simulink model "CarWashSimulinkSimulator"  (R2021b)
settings: Solver=FixedStepDiscrete  StartTime=0.0  StopTime=inf  RelTol=1e-3
model workspace (MAT data in the model file):
  SoapLevel = Simulink.Parameter
  SoapLevel.Value = 100
  SoapLevel.DataType = 'int8'
  SoapLevel.Min = 0
  SoapLevel.Max = 100
  SoapLevel.Complexity = 'real'
  SoapLevel.Dimensions = [1 1]
  UltraShineLevel = Simulink.Parameter
  UltraShineLevel.Value = 100
  UltraShineLevel.DataType = 'int8'
  UltraShineLevel.Min = 0
  UltraShineLevel.Max = 100
  UltraShineLevel.Complexity = 'real'
  UltraShineLevel.Dimensions = [1 1]
  WashType = 'standard'
  WaterPumpStatus = 1
  WaxLevel = Simulink.Parameter
  WaxLevel.Value = 1
  WaxLevel.DataType = 'double'
  WaxLevel.Min = 0
  WaxLevel.Max = 100
  WaxLevel.Complexity = 'real'
  WaxLevel.Dimensions = [1 1]
settings Model: Creator=Daniel Hernandez  LastModifiedBy=Daniel Hernandez

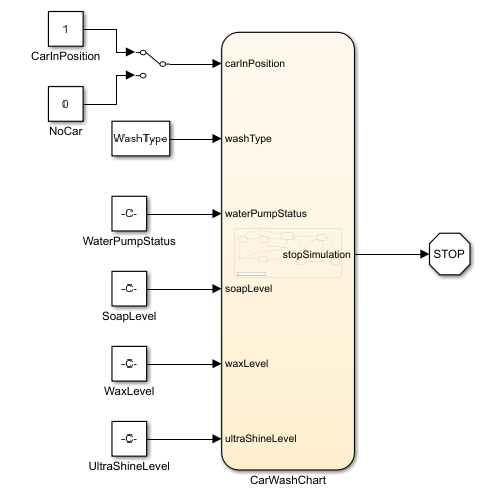
[thumbnail: Simulink's stored preview of the top-level diagram]
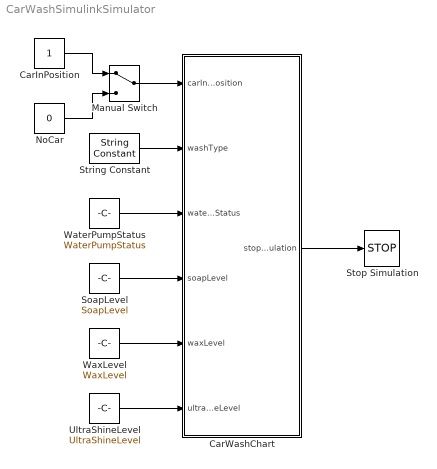
== system CarWashSimulinkSimulator ==
  CarInPosition : Constant
  CarWashChart : Stateflow chart  TreatAsAtomicUnit=on
  Manual Switch : ManualSwitch
  NoCar : Constant  Value=0
  SoapLevel : Constant  Value=SoapLevel
  Stop Simulation : Stop
  String Constant : StringConstant  String=WashType
  UltraShineLevel : Constant  Value=UltraShineLevel
  WaterPumpStatus : Constant  Value=WaterPumpStatus
  WaxLevel : Constant  Value=WaxLevel
  wires:
  CarInPosition/1 -> Manual Switch/1
  NoCar/1 -> Manual Switch/2
  Manual Switch/1 -> CarWashChart/1(carInPosition)
  CarWashChart/1(stopSimulation) -> Stop Simulation/1
  String Constant/1 -> CarWashChart/2(washType)
  WaterPumpStatus/1 -> CarWashChart/3(waterPumpStatus)
  SoapLevel/1 -> CarWashChart/4(soapLevel)
  WaxLevel/1 -> CarWashChart/5(waxLevel)
  UltraShineLevel/1 -> CarWashChart/6(ultraShineLevel)

== stateflow chart CarWashSimulinkSimulator/CarWashChart ==
  state AppInterface
    state Idle
    state Exiting
      ex:
      stopSimulation = 1
    state Ready
    state SprayingWater
    state Drying
    state Foaming
    state Waxing
    state Polishing
    state ValidationFailed
    (default) -> Idle
    Ready -> Exiting [order 2] : after(10,sec)
    Exiting -> Idle
    ValidationFailed -> Exiting
    (junction 26) -> Exiting [order 1] : [washType=='quick']
    (junction 30) -> Exiting [order 4]
    Drying -> Exiting : after(5,sec)
    Idle -> Ready [order 1] : after(1,sec)
    Ready -> (junction 25) [order 1] : [carInPosition == true]
    (junction 25) -> SprayingWater [order 1] : [washType=='quick']
    (junction 25) -> Foaming [order 2] : [washType~='quick']
    Idle -> ValidationFailed [order 2] : [~canStartWash(waterPumpStatus, soapLevel)]
    Foaming -> SprayingWater : after(5,sec)
    SprayingWater -> (junction 26) : after(5,sec)
    (junction 26) -> Drying [order 2] : [washType=='standard']
    (junction 30) -> Drying [order 1] : [washType~='ultimate']
    (junction 26) -> ValidationFailed [order 4] : [waxLevel < 5 & washType=='standard' ]
    Polishing -> Drying : after(5,sec)
    (junction 26) -> Waxing [order 3] : [isequal(washType,'premium') || isequal(washType,'ultimate')]
    Waxing -> (junction 30) : after(5,sec)
    (junction 30) -> Polishing [order 2] : [washType=='ultimate']
    (junction 30) -> ValidationFailed [order 3] : [washType=='ultimate' & ultraShineLevel < 5]
  (default) -> AppInterface
  data: pumpStatus function_input; soapLvl function_input; result function_output; carInPosition input; stopSimulation output =0; washType input; waterPumpStatus input; soapLevel input; waxLevel input; ultraShineLevel input
  function result = canStartWash (pumpStatus, soapLvl):
    | function result = canStartWash (pumpStatus, soapLvl)
    |     if(pumpStatus == 0)
    |         result = false;
    |     else if (soapLvl < 10)
    |         result = false;
    |     else
    |         result = true;
    |     end
    | end
